simulink library "ddm"  (R2021b)
settings: Solver=VariableStepAuto  StartTime=0.0  StopTime=10.0  RelTol=1e-3
undefined symbols (not defined in the file or in its folder): ENUM_ADASACCSTA_ERROR, ENUM_ADASACCSTA_OFF, ENUM_ADASACCSTA_STANDBY, ENUM_ADASISASTA_OFF, ENUM_ALLOWMOV_ALLOWREADY, ENUM_APS, ENUM_BRKSTA_ERROR, ENUM_BRKSTA_OFF, ENUM_BRKSTA_ON, ENUM_BRKSW_INVALID, ENUM_BRKSW_OFF, ENUM_BRKSW_ON, ENUM_CHGPREACTERRSTA_OBCPRE, ENUM_DCDCFAULTSTA_ANYFAULTLV1, ENUM_DCDCFAULTSTA_ANYFAULTLV2, ENUM_DRIVETRAIN_AWD, ENUM_DRIVETRAIN_FWD, ENUM_DRIVETRAIN_RWD, ENUM_DRSEATSTA_INVALID, ENUM_EDUDRTSTA_NORMAL, ENUM_EPBSTA_APPLIED, ENUM_EPBSTA_RELEASED, ENUM_HVBATTREADYPRE_READY, ENUM_MCUWARN_LV0, ENUM_MCUWARN_LV1, ENUM_MCUWARN_LV2, ENUM_MCUWARN_LV3, ENUM_MCUWARN_NOERROR, ENUM_OBCFAULTSTA_ANYFAULT, ENUM_PAS_R2F2, ENUM_PDFAULT_BATTPDFAIL, ENUM_PDFAULT_DCDCDISABLE, ENUM_PDFAULT_MCUDISABLE, ENUM_PDFAULT_MCUDISCHRG, ENUM_POWERSTA_OFF, ENUM_POWERSTA_ON, ENUM_POWERSTA_READY, ENUM_POWERSTA_STANDBY, ENUM_PRESSINDI_LOW, ENUM_PUFAULT_BATTUPFAIL, ENUM_PUFAULT_DCDCENABLEFAIL, ENUM_PUFAULT_PRECHRGCHKFAIL, ENUM_PUFAULT_SAFETYCHKFAIL, ENUM_PUSTATE_COMPLETED, ENUM_PWRSTASW_OFF, ENUM_PWRSTASW_OFFA, ENUM_PWRSTASW_OFFCHVCHRG, ENUM_PWRSTASW_OFFCLVCHRG, ENUM_PWRSTASW_ON, ENUM_PWRSTASW_ONHVCHRG, ENUM_PWRSTASW_READY, ENUM_PWRSTASW_STANDBY, ENUM_RANGESTA_12IN, ENUM_SHIFTCOMMAND_D, ENUM_SHIFTCOMMAND_N, ENUM_SHIFTCOMMAND_P, ENUM_SHIFTCOMMAND_R, ENUM_VEHMALFUNLV_2ND, ENUM_VEHMALFUNLV_3RD, ENUM_VEHMALFUNLV_4TH ... (+835)
libraries: hcu_lib x750, $bdroot x12, simulink x5
(part 23 of 28)

== system ddm/DDM/DDM/VMC_DDM/ACC Acceleration Command Error/ACC Acceleration Command Error  ==
  note: Diagnostics and Fault Handling
  note: Fail Safe After Decision
  note: Release Condiction During Detection
  note: Release Condiction After Decision
  note: Test Pass Criteria
  note: Test Detection Criteria
  note: Fail Safe During Detection
  task_time_s : Inport
  VDDM_FCM2NoComCFS_flg : Inport  Port=2
  VDDM_FCM2RCErrCFS_flg : Inport  Port=3
  VDDM_FCM2CSErrCFS_flg : Inport  Port=4
  VVMC_ADASActive_flg : Inport  Port=5
  No_CAN_BUS_OFF : Inport  Port=6
  VPMM_PowerSta_enum : Inport  Port=7
  VINP_ACCRequireAccel_mps2 : Inport  Port=8
  VINP_ADASACCSta_enum : Inport  Port=9
  DTC_clear_request : Inport  Port=10
  Abs : Abs
  Abs1 : Abs
  Constant1 : Constant  Value=KDDM_ACCAccelCmdErrDet_mps2
  Constant10 : Constant  Value=ENUM_ADASACCSTA_OFF
  Constant11 : Constant  Value=KDDM_ACCAccelCmdErrPassSW_flg
  Constant12 : Constant  Value=ENUM_POWERSTA_OFF
  Constant13 : Constant  Value=ENUM_POWERSTA_STANDBY
  Constant{5,14,18,22} (4 alike) : Constant  Value=TRUE
  Constant{2,15..16,21,23} (5 alike) : Constant  Value=FALSE
  Constant3 : Constant  Value=KDDM_ACCAccelCmdErrDet_mps2
  Constant33 : Constant  Value=KDDM_ACCAccelCmdErrDetSW_flg
  Constant34 : Constant  Value=KDDM_ACCAccelCmdErrDTC_cnt
  Constant35 : Constant  Value=KDDM_ACCAccelCmdErrCFSSW_flg
  Constant36 : Constant  Value=KDDM_ACCAccelCmdErrDFSSW_flg
  Constant4 : Constant  Value=KDDM_ACCAccelCmdErrDetTO_ms
  Constant6 : Constant  Value=KDDM_ACCAccelCmdErrPassTO_ms
  Constant7 : Constant  Value=KDDM_ACCAccelCmdErrDTC_cnt
  Constant8 : Constant  Value=ENUM_ADASACCSTA_STANDBY
  Constant9 : Constant  Value=KDDM_ACCAccelCmdErrPassTO_ms
  DTC_Couter : hcu_lib/Basic_Blocks/DTC_Couter
  DTC_Info : hcu_lib/Basic_Blocks/DTC_Info
  Data Type Conversion1 : DataTypeConversion  OutDataTypeStr=uint8
  Equal1 : RelationalOperator  Operator=>  OutDataTypeStr=boolean  RndMeth=Simplest
  Equal2 : RelationalOperator  Operator=>  OutDataTypeStr=boolean  RndMeth=Simplest
  Equal3 : RelationalOperator  OutDataTypeStr=boolean  RndMeth=Simplest
  Equal{4..7} (4 alike) : RelationalOperator  Operator===  OutDataTypeStr=boolean  RndMeth=Simplest
  From1 : From  Commented=on  GotoTag=VDDM_ACCAccelCmdErrDFS_flg
  Gain : Gain  Gain=XX2KXX
  Gain1 : Gain  Gain=KXX2XX
  Goto7 : Goto  Commented=on  GotoTag=VDDM_EDriveSysErrVCUErr_flg
  Logical Operator{1,4,6,11,14,17..18,20} (8 alike) : Logic  Operator=NOT  AllPortsSameDT=off  OutDataTypeStr=boolean
  Logical Operator10 : Logic  Inputs=5  AllPortsSameDT=off  OutDataTypeStr=boolean
  Logical Operator12 : Logic  Operator=OR  Inputs=3  AllPortsSameDT=off  OutDataTypeStr=boolean
  Logical Operator{3,5,8,13,15} (5 alike) : Logic  AllPortsSameDT=off  OutDataTypeStr=boolean
  Logical Operator16 : Logic  Operator=OR  AllPortsSameDT=off  OutDataTypeStr=boolean
  Logical Operator19 : Logic  Inputs=3  AllPortsSameDT=off  OutDataTypeStr=boolean
  Logical Operator2 : Logic  Inputs=5  AllPortsSameDT=off  OutDataTypeStr=boolean
  Logical Operator25 : Logic  Operator=OR  Inputs=3  AllPortsSameDT=off  OutDataTypeStr=boolean
  Logical Operator7 : Logic  Operator=OR  Inputs=3  AllPortsSameDT=off  OutDataTypeStr=boolean
  Logical Operator9 : Logic  Operator=OR  AllPortsSameDT=off  OutDataTypeStr=boolean
  Relay : Relay  OnSwitchValue=ONE_INT  OffSwitchValue=ZERO_INT
  SR_Latch1 : hcu_lib/Basic_Blocks/SR_Latch
  SR_Latch4 : hcu_lib/Basic_Blocks/SR_Latch
  SR_Latch5 : hcu_lib/Basic_Blocks/SR_Latch
  Switch{,1..5} (6 alike) : Switch  Criteria=u2 ~= 0
  Terminator1 : Terminator
  Test Detection Criteria : hcu_lib/Basic_Blocks/Test Detection Criteria
  Timer1 : hcu_lib/Basic_Blocks/Timer
  Unit Delay2 : UnitDelay  SampleTime=-1  HasFrameUpgradeWarning=on
  VDDM_ACCAccelCmdErrCFS_flg : Outport
  VDDM_ACCAccelCmdErrDetDTC_raw32 : Outport  Port=2
  wires:
  Constant11/1 -> Logical Operator15/2
  DTC_Couter/1 -> SR_Latch5/1
  SR_Latch4/1 -> Logical Operator3/2
  Logical Operator25/1 -> Logical Operator15/1
  SR_Latch5/1 -> Logical Operator5/1
  Data Type Conversion1/1 -> [VDDM_ACCAccelCmdErrDTC_cnt]  "VDDM_ACCAccelCmdErrDTC_cnt"
  Constant36/1 -> Logical Operator3/1
  Relay/1 -> SR_Latch4/1
  [VDDM_ACCAccelCmdErrCFS_flg] -> Logical Operator7/2
  [VDDM_ACCAccelCmdErrDFSRls_flg] -> Logical Operator7/1
  [DTC_clear_request] -> Logical Operator25/1, Logical Operator14/1
  Constant33/1 -> Logical Operator19/2
  Logical Operator5/1 -> [VDDM_ACCAccelCmdErrCFS_flg]  "VDDM_ACCAccelCmdErrCFS_flg"
  Logical Operator3/1 -> [VDDM_ACCAccelCmdErrDFS_flg]
  [VDDM_ACCAccelCmdErrCFSRls_flg] -> Logical Operator25/3
  [VDDM_ACCAccelCmdErrPass_flg] -> Logical Operator25/2
  [VDDM_ACCAccelCmdErrDet_flg] -> Logical Operator19/1
  [DTC_clear_request] -> Logical Operator7/3
  Logical Operator16/1 -> SR_Latch5/2
  [DTC_clear_request] -> Logical Operator16/2
  Logical Operator14/1 -> Logical Operator19/3
  [VDDM_ACCAccelCmdErrCFSRls_flg] -> Logical Operator16/1
  [VDDM_ACCAccelCmdErrDTC_cnt] -> Relay/1
  Logical Operator15/1 -> DTC_Couter/2
  Logical Operator19/1 -> DTC_Couter/1
  Constant35/1 -> Logical Operator5/2
  Constant34/1 -> DTC_Couter/3
  DTC_Couter/2 -> Data Type Conversion1/1
  Logical Operator7/1 -> SR_Latch4/2
  DTC_Info/1 -> VDDM_ACCAccelCmdErrDetDTC_raw32/1  "VDDM_ACCAccelCmdErrDetDTC_raw32"
  [DTC_clear_request] -> DTC_Info/4
  [VDDM_ACCAccelCmdErrCFS_flg] -> DTC_Info/3
  [VDDM_ACCAccelCmdErrPass_flg] -> DTC_Info/2
  [VDDM_ACCAccelCmdErrDet_flg] -> DTC_Info/1
  [DTC_clear_request] -> Switch5/2
  Constant16/1 -> Switch5/1
  Switch5/1 -> Test Detection Criteria/1
  VINP_ADASACCSta_enum/1 -> [VINP_ADASACCSta_enum]
  [VDDM_ACCAccelCmdErrPass_flg] -> Logical Operator8/1
  Constant12/1 -> Equal6/2
  Equal5/1 -> Logical Operator9/2
  [VINP_ADASACCSta_enum] -> Equal4/1
  [VINP_ADASACCSta_enum] -> Equal5/1
  Constant13/1 -> Equal7/2
  Logical Operator8/1 -> Logical Operator12/1
  Equal4/1 -> Logical Operator9/1
  Equal6/1 -> Logical Operator13/1
  Logical Operator13/1 -> Logical Operator12/2
  Equal7/1 -> Logical Operator13/2
  Unit Delay2/1 -> Equal6/1
  Constant10/1 -> Equal4/2
  Logical Operator9/1 -> Logical Operator8/2
  Constant8/1 -> Equal5/2
  [VPMM_PowerSta_enum] -> Equal7/1
  [VPMM_PowerSta_enum] -> Unit Delay2/1
  [VDDM_FCM2NoComCFS_flg] -> Logical Operator1/1
  Abs1/1 -> Equal1/1
  [No_CAN_BUS_OFF] -> Logical Operator10/1
  [VDDM_FCM2CSErrCFS_flg] -> Logical Operator11/1
  Logical Operator10/1 -> Switch3/2
  Constant1/1 -> Equal1/2
  [VVMC_ADASActive_flg] -> Logical Operator10/5
  Equal1/1 -> Switch3/1
  Logical Operator4/1 -> Logical Operator10/3
  [VINP_ACCRequireAccel_mps2] -> Abs1/1
  Logical Operator11/1 -> Logical Operator10/4
  [VDDM_FCM2RCErrCFS_flg] -> Logical Operator4/1
  Logical Operator1/1 -> Logical Operator10/2
  Abs/1 -> Equal2/1
  VVMC_ADASActive_flg/1 -> [VVMC_ADASActive_flg]
  Equal2/1 -> Switch2/1
  Constant3/1 -> Equal2/2
  Constant9/1 -> Timer1/4
  Gain1/1 -> Timer1/3
  Test Detection Criteria/1 -> [VDDM_ACCAccelCmdErrDet_flg]  "VDDM_ACCAccelCmdErrDet_flg"
  Constant7/1 -> Test Detection Criteria/3
  Gain/1 -> Test Detection Criteria/4
  Constant4/1 -> Gain/1
  [task_time_s] -> Test Detection Criteria/2
  task_time_s/1 -> [task_time_s]  "task_time_s"
  Switch3/1 -> Logical Operator6/1, Timer1/2
  Constant5/1 -> Switch3/3
  Logical Operator20/1 -> Logical Operator2/4
  Logical Operator18/1 -> Logical Operator2/3
  Logical Operator17/1 -> Logical Operator2/2
  [VINP_ACCRequireAccel_mps2] -> Abs/1
  [VDDM_FCM2CSErrCFS_flg] -> Logical Operator20/1
  [VDDM_FCM2RCErrCFS_flg] -> Logical Operator18/1
  [VDDM_FCM2NoComCFS_flg] -> Logical Operator17/1
  [VVMC_ADASActive_flg] -> Logical Operator2/5
  VINP_ACCRequireAccel_mps2/1 -> [VINP_ACCRequireAccel_mps2]
  No_CAN_BUS_OFF/1 -> [No_CAN_BUS_OFF]
  VDDM_FCM2CSErrCFS_flg/1 -> [VDDM_FCM2CSErrCFS_flg]
  VPMM_PowerSta_enum/1 -> [VPMM_PowerSta_enum]
  VDDM_FCM2RCErrCFS_flg/1 -> [VDDM_FCM2RCErrCFS_flg]
  DTC_clear_request/1 -> [DTC_clear_request]
  VDDM_FCM2NoComCFS_flg/1 -> [VDDM_FCM2NoComCFS_flg]
  Timer1/1 -> Equal3/1
  Logical Operator12/1 -> Switch4/2
  Constant14/1 -> Switch4/1
  Constant2/1 -> Switch2/3
  Logical Operator6/1 -> Timer1/1
  Logical Operator2/1 -> Switch2/2
  [DTC_clear_request] -> Logical Operator12/3
  [VDDM_xxx_flg] -> SR_Latch1/2
  [No_CAN_BUS_OFF] -> Logical Operator2/1
  Switch4/1 -> [VDDM_ACCAccelCmdErrCFSRls_flg]  "VDDM_ACCAccelCmdErrCFSRls_flg"
  Constant6/1 -> Equal3/2
  [task_time_s] -> Gain1/1
  Equal3/1 -> SR_Latch1/1
  Constant15/1 -> Switch4/3
  [VDDM_ACCAccelCmdErrCFS_flg] -> VDDM_ACCAccelCmdErrCFS_flg/1
  From1/1 -> Terminator1/1
  SR_Latch1/1 -> [VDDM_ACCAccelCmdErrPass_flg]  "VDDM_ACCAccelCmdErrPass_flg"
  [VDDM_ACCAccelCmdErrPass_flg] -> Switch1/2
  [VDDM_ACCAccelCmdErrCFS_flg] -> Switch/2
  Constant18/1 -> Switch/1
  Switch/1 -> Goto7/1
  Constant21/1 -> Switch/3
  Switch1/1 -> [VDDM_ACCAccelCmdErrDFSRls_flg]
  Constant22/1 -> Switch1/1
  Constant23/1 -> Switch1/3
  Switch2/1 -> Switch5/3, [VDDM_xxx_flg]

== system ddm/DDM/DDM/VMC_DDM/ACC Malfunction /ACC Malfunction  ==
  note: Diagnostics and Fault Handling
  note: Fail Safe After Decision
  note: Release Condiction During Detection
  note: Release Condiction After Decision
  note: Test Pass Criteria
  note: Test Detection Criteria
  note: Fail Safe During Detection
  task_time_s : Inport
  VDDM_FCMACCSigErrCFS_flg : Inport  Port=2
  VDDM_ACCAccelCmdErrCFS_flg : Inport  Port=3
  VDDM_BMSSigErrCFS_flg : Inport  Port=4
  VDDM_FrMCUSigErrCFS_flg : Inport  Port=5
  VDDM_RrMCUSigErrCFS_flg : Inport  Port=6
  VDDM_CCUSigErrCFS_flg : Inport  Port=7
  VDDM_FCM2NoComCFS_flg : Inport  Port=8
  VDDM_FCM2RCErrCFS_flg : Inport  Port=9
  VDDM_FCM2CSErrCFS_flg : Inport  Port=10
  VDDM_FCM4NoComCFS_flg : Inport  Port=11
  VDDM_FCM4CSErrCFS_flg : Inport  Port=12
  VDDM_ZoneSCPNoComCFS_flg : Inport  Port=13
  VDDM_MCUR1NoComCFS_flg : Inport  Port=14
  VDDM_MCUR1RCErrCFS_flg : Inport  Port=15
  VDDM_MCUR1CSErrCFS_flg : Inport  Port=16
  VDDM_MCUF1NoComCFS_flg : Inport  Port=17
  VDDM_MCUF1RCErrCFS_flg : Inport  Port=18
  VDDM_MCUF1CSErrCFS_flg : Inport  Port=19
  VDDM_ESC7NoComCFS_flg : Inport  Port=20
  VDDM_ESC7RCErrCFS_flg : Inport  Port=21
  VDDM_ESC7CSErrCFS_flg : Inport  Port=22
  VDDM_ESC1NoComCFS_flg : Inport  Port=23
  VDDM_ESC1RCErrCFS_flg : Inport  Port=24
  VDDM_ESC1CSErrCFS_flg : Inport  Port=25
  VDDM_ESC5NoComCFS_flg : Inport  Port=26
  VDDM_ESC5RCErrCFS_flg : Inport  Port=27
  VDDM_ESC5CSErrCFS_flg : Inport  Port=28
  No_CAN1_BUS_OFF : Inport  Port=29
  No_CAN3_BUS_OFF : Inport  Port=30
  No_CAN4_BUS_OFF : Inport  Port=31
  VPMM_PowerSta_enum : Inport  Port=32
  VINP_ZoneSpdCtrlMode_enum : Inport  Port=33
  DTC_clear_request : Inport  Port=34
  Constant1 : Constant  Value=ENUM_POWERSTA_READY
  Constant10 : Constant  Value=ENUM_ZONESPDCTRLMODE_ACC
  Constant11 : Constant  Value=KDDM_ACCMalfuncPassSW_flg
  Constant12 : Constant  Value=ENUM_POWERSTA_OFF
  Constant13 : Constant  Value=ENUM_POWERSTA_STANDBY
  Constant{5,14,18,22} (4 alike) : Constant  Value=TRUE
  Constant{2,15..16,21,23} (5 alike) : Constant  Value=FALSE
  Constant3 : Constant  Value=ENUM_ZONESPDCTRLMODE_ACC
  Constant33 : Constant  Value=KDDM_ACCMalfuncDetSW_flg
  Constant34 : Constant  Value=KDDM_ACCMalfuncDTC_cnt
  Constant35 : Constant  Value=KDDM_ACCMalfuncCFSSW_flg
  Constant36 : Constant  Value=KDDM_ACCMalfuncDFSSW_flg
  Constant4 : Constant  Value=KDDM_ACCMalfuncDetTO_ms
  Constant6 : Constant  Value=KDDM_ACCMalfuncPassTO_ms
  Constant7 : Constant  Value=KDDM_ACCMalfuncDTC_cnt
  Constant8 : Constant  Value=ENUM_POWERSTA_READY
  Constant9 : Constant  Value=KDDM_ACCMalfuncPassTO_ms
  DTC_Couter : hcu_lib/Basic_Blocks/DTC_Couter
  DTC_Info : hcu_lib/Basic_Blocks/DTC_Info
  Data Type Conversion1 : DataTypeConversion  OutDataTypeStr=uint8
  Equal{1..2,4..7} (6 alike) : RelationalOperator  Operator===  OutDataTypeStr=boolean  RndMeth=Simplest
  Equal3 : RelationalOperator  OutDataTypeStr=boolean  RndMeth=Simplest
  From1 : From  Commented=on  GotoTag=VDDM_ACCMalfuncDFS_flg
  Gain : Gain  Gain=XX2KXX
  Gain1 : Gain  Gain=KXX2XX
  Goto7 : Goto  Commented=on  GotoTag=VDDM_EDriveSysErrVCUErr_flg
  Logical Operator1 : Logic  Inputs=5  AllPortsSameDT=off  OutDataTypeStr=boolean
  Logical Operator12 : Logic  Operator=OR  Inputs=3  AllPortsSameDT=off  OutDataTypeStr=boolean
  Logical Operator{3,5,13,15} (4 alike) : Logic  AllPortsSameDT=off  OutDataTypeStr=boolean
  Logical Operator14 : Logic  Operator=OR  Inputs=27  AllPortsSameDT=off  OutDataTypeStr=boolean
  Logical Operator19 : Logic  Inputs=3  AllPortsSameDT=off  OutDataTypeStr=boolean
  Logical Operator2 : Logic  Inputs=5  AllPortsSameDT=off  OutDataTypeStr=boolean
  Logical Operator25 : Logic  Operator=OR  Inputs=3  AllPortsSameDT=off  OutDataTypeStr=boolean
  Logical Operator4 : Logic  Operator=OR  Inputs=27  AllPortsSameDT=off  OutDataTypeStr=boolean
  Logical Operator6 : Logic  Operator=NOT  AllPortsSameDT=off  OutDataTypeStr=boolean
  Logical Operator7 : Logic  Operator=OR  Inputs=3  AllPortsSameDT=off  OutDataTypeStr=boolean
  Logical Operator8 : Logic  Operator=NOT  AllPortsSameDT=off  OutDataTypeStr=boolean
  Logical Operator9 : Logic  Operator=OR  AllPortsSameDT=off  OutDataTypeStr=boolean
  Relay : Relay  OnSwitchValue=ONE_INT  OffSwitchValue=ZERO_INT
  SR_Latch1 : hcu_lib/Basic_Blocks/SR_Latch
  SR_Latch4 : hcu_lib/Basic_Blocks/SR_Latch
  SR_Latch5 : hcu_lib/Basic_Blocks/SR_Latch
  Switch{,1..5} (6 alike) : Switch  Criteria=u2 ~= 0
  Terminator1 : Terminator
  Test Detection Criteria : hcu_lib/Basic_Blocks/Test Detection Criteria
  Timer1 : hcu_lib/Basic_Blocks/Timer
  Unit Delay2 : UnitDelay  SampleTime=-1  HasFrameUpgradeWarning=on
  VDDM_ACCMalfuncCFS_flg : Outport
  VDDM_ACCMalfuncDetDTC_raw32 : Outport  Port=2
  wires:
  [VDDM_ACCMalfuncDFSRls_flg] -> Logical Operator7/1
  Logical Operator8/1 -> Logical Operator19/3
  [DTC_clear_request] -> Logical Operator9/2
  Logical Operator5/1 -> [VDDM_ACCMalfuncCFS_flg]  "VDDM_ACCMalfuncCFS_flg"
  [DTC_clear_request] -> Logical Operator25/1, Logical Operator8/1
  [VDDM_ACCMalfuncCFSRls_flg] -> Logical Operator25/3
  Logical Operator9/1 -> SR_Latch5/2
  [VDDM_ACCMalfuncCFS_flg] -> Logical Operator7/2
  [VDDM_ACCMalfuncDTC_cnt] -> Relay/1
  [DTC_clear_request] -> Logical Operator7/3
  Constant35/1 -> Logical Operator5/2
  Constant33/1 -> Logical Operator19/2
  Logical Operator19/1 -> DTC_Couter/1
  SR_Latch5/1 -> Logical Operator5/1
  Relay/1 -> SR_Latch4/1
  Constant34/1 -> DTC_Couter/3
  Logical Operator25/1 -> Logical Operator15/1
  [VDDM_ACCMalfuncDet_flg] -> Logical Operator19/1
  Data Type Conversion1/1 -> [VDDM_ACCMalfuncDTC_cnt]  "VDDM_ACCMalfuncDTC_cnt"
  DTC_Couter/2 -> Data Type Conversion1/1
  Logical Operator7/1 -> SR_Latch4/2
  Constant36/1 -> Logical Operator3/1
  SR_Latch4/1 -> Logical Operator3/2
  [VDDM_ACCMalfuncCFSRls_flg] -> Logical Operator9/1
  Logical Operator15/1 -> DTC_Couter/2
  Logical Operator3/1 -> [VDDM_ACCMalfuncDFS_flg]
  [VDDM_ACCMalfuncPass_flg] -> Logical Operator25/2
  Constant11/1 -> Logical Operator15/2
  DTC_Couter/1 -> SR_Latch5/1
  DTC_Info/1 -> VDDM_ACCMalfuncDetDTC_raw32/1  "VDDM_ACCMalfuncDetDTC_raw32"
  [DTC_clear_request] -> DTC_Info/4
  [VDDM_ACCMalfuncCFS_flg] -> DTC_Info/3
  [VDDM_ACCMalfuncPass_flg] -> DTC_Info/2
  [VDDM_ACCMalfuncDet_flg] -> DTC_Info/1
  [DTC_clear_request] -> Switch5/2
  Constant16/1 -> Switch5/1
  Switch5/1 -> Test Detection Criteria/1
  [VDDM_ESC5NoComCFS_flg] -> Logical Operator4/25
  [VDDM_MCUF1RCErrCFS_flg] -> Logical Operator4/17
  [VDDM_ESC5RCErrCFS_flg] -> Logical Operator4/26
  [VDDM_MCUR1RCErrCFS_flg] -> Logical Operator4/14
  [VDDM_ESC5CSErrCFS_flg] -> Logical Operator4/27
  [VDDM_MCUF1NoComCFS_flg] -> Logical Operator4/16
  [VDDM_MCUR1CSErrCFS_flg] -> Logical Operator4/15
  [VDDM_ESC1RCErrCFS_flg] -> Logical Operator4/23
  [VDDM_ESC7NoComCFS_flg] -> Logical Operator4/19
  [VDDM_FrMCUSigErrCFS_flg] -> Logical Operator4/4
  [VDDM_MCUF1CSErrCFS_flg] -> Logical Operator4/18
  [VDDM_RrMCUSigErrCFS_flg] -> Logical Operator4/5
  [VDDM_ESC7RCErrCFS_flg] -> Logical Operator4/20
  [VDDM_FCM4CSErrCFS_flg] -> Logical Operator4/11
  [VDDM_ESC7CSErrCFS_flg] -> Logical Operator4/21
  [VDDM_MCUR1NoComCFS_flg] -> Logical Operator4/13
  [VDDM_ESC1NoComCFS_flg] -> Logical Operator4/22
  [VDDM_ESC1CSErrCFS_flg] -> Logical Operator4/24
  Logical Operator4/1 -> Switch3/1
  [VDDM_ACCAccelCmdErrCFS_flg] -> Logical Operator4/2
  [VDDM_BMSSigErrCFS_flg] -> Logical Operator4/3
  [VDDM_CCUSigErrCFS_flg] -> Logical Operator4/6
  [VDDM_FCM2NoComCFS_flg] -> Logical Operator4/7
  [VDDM_FCM2RCErrCFS_flg] -> Logical Operator4/8
  [VDDM_FCM4NoComCFS_flg] -> Logical Operator4/10
  [VDDM_FCM2CSErrCFS_flg] -> Logical Operator4/9
  [VDDM_ZoneSCPNoComCFS_flg] -> Logical Operator4/12
  [VDDM_FCMACCSigErrCFS_flg] -> Logical Operator4/1
  Logical Operator1/1 -> Switch3/2
  [No_CAN1_BUS_OFF] -> Logical Operator1/1
  [No_CAN3_BUS_OFF] -> Logical Operator1/2
  Equal4/1 -> Logical Operator1/5
  Equal5/1 -> Logical Operator1/4
  Constant8/1 -> Equal5/2
  Constant10/1 -> Equal4/2
  [VPMM_PowerSta_enum] -> Equal5/1
  [No_CAN4_BUS_OFF] -> Logical Operator1/3
  [VINP_ZoneSpdCtrlMode_enum] -> Equal4/1
  Equal1/1 -> Logical Operator2/5
  Constant3/1 -> Equal1/2
  [VINP_ZoneSpdCtrlMode_enum] -> Equal1/1
  [VPMM_PowerSta_enum] -> Equal2/1
  Constant1/1 -> Equal2/2
  Equal2/1 -> Logical Operator2/4
  [No_CAN4_BUS_OFF] -> Logical Operator2/3
  [No_CAN3_BUS_OFF] -> Logical Operator2/2
  Logical Operator14/1 -> Switch2/1
  [VDDM_ESC5CSErrCFS_flg] -> Logical Operator14/27
  [VDDM_ESC5RCErrCFS_flg] -> Logical Operator14/26
  [VDDM_ESC5NoComCFS_flg] -> Logical Operator14/25
  [VDDM_ESC1CSErrCFS_flg] -> Logical Operator14/24
  [VDDM_ESC1RCErrCFS_flg] -> Logical Operator14/23
  [VDDM_ESC1NoComCFS_flg] -> Logical Operator14/22
  [VDDM_ESC7CSErrCFS_flg] -> Logical Operator14/21
  [VDDM_ESC7RCErrCFS_flg] -> Logical Operator14/20
  [VDDM_ESC7NoComCFS_flg] -> Logical Operator14/19
  [VDDM_MCUF1CSErrCFS_flg] -> Logical Operator14/18
  [VDDM_MCUF1RCErrCFS_flg] -> Logical Operator14/17
  [VDDM_MCUF1NoComCFS_flg] -> Logical Operator14/16
  [VDDM_MCUR1CSErrCFS_flg] -> Logical Operator14/15
  [VDDM_MCUR1RCErrCFS_flg] -> Logical Operator14/14
  [VDDM_MCUR1NoComCFS_flg] -> Logical Operator14/13
  [VDDM_ZoneSCPNoComCFS_flg] -> Logical Operator14/12
  [VDDM_FCM4CSErrCFS_flg] -> Logical Operator14/11
  [VDDM_FCM4NoComCFS_flg] -> Logical Operator14/10
  [VDDM_FCM2CSErrCFS_flg] -> Logical Operator14/9
  [VDDM_FCM2RCErrCFS_flg] -> Logical Operator14/8
  [VDDM_FCM2NoComCFS_flg] -> Logical Operator14/7
  [VDDM_CCUSigErrCFS_flg] -> Logical Operator14/6
  [VDDM_RrMCUSigErrCFS_flg] -> Logical Operator14/5
  [VDDM_FrMCUSigErrCFS_flg] -> Logical Operator14/4
  [VDDM_BMSSigErrCFS_flg] -> Logical Operator14/3
  [VDDM_ACCAccelCmdErrCFS_flg] -> Logical Operator14/2
  [VDDM_FCMACCSigErrCFS_flg] -> Logical Operator14/1
  VDDM_ESC5RCErrCFS_flg/1 -> [VDDM_ESC5RCErrCFS_flg]
  VDDM_ACCAccelCmdErrCFS_flg/1 -> [VDDM_ACCAccelCmdErrCFS_flg]
  VDDM_ESC5CSErrCFS_flg/1 -> [VDDM_ESC5CSErrCFS_flg]
  VDDM_ESC5NoComCFS_flg/1 -> [VDDM_ESC5NoComCFS_flg]
  VDDM_ZoneSCPNoComCFS_flg/1 -> [VDDM_ZoneSCPNoComCFS_flg]
  task_time_s/1 -> [task_time_s]  "task_time_s"
  VINP_ZoneSpdCtrlMode_enum/1 -> [VINP_ZoneSpdCtrlMode_enum]
  No_CAN3_BUS_OFF/1 -> [No_CAN3_BUS_OFF]
  No_CAN1_BUS_OFF/1 -> [No_CAN1_BUS_OFF]
  VDDM_BMSSigErrCFS_flg/1 -> [VDDM_BMSSigErrCFS_flg]
  VDDM_ESC7NoComCFS_flg/1 -> [VDDM_ESC7NoComCFS_flg]
  VDDM_FCMACCSigErrCFS_flg/1 -> [VDDM_FCMACCSigErrCFS_flg]
  VDDM_ESC7CSErrCFS_flg/1 -> [VDDM_ESC7CSErrCFS_flg]
  VPMM_PowerSta_enum/1 -> [VPMM_PowerSta_enum]
  No_CAN4_BUS_OFF/1 -> [No_CAN4_BUS_OFF]
  VDDM_ESC7RCErrCFS_flg/1 -> [VDDM_ESC7RCErrCFS_flg]
  VDDM_RrMCUSigErrCFS_flg/1 -> [VDDM_RrMCUSigErrCFS_flg]
  VDDM_CCUSigErrCFS_flg/1 -> [VDDM_CCUSigErrCFS_flg]
  VDDM_FrMCUSigErrCFS_flg/1 -> [VDDM_FrMCUSigErrCFS_flg]
  VDDM_MCUF1RCErrCFS_flg/1 -> [VDDM_MCUF1RCErrCFS_flg]
  VDDM_ESC1NoComCFS_flg/1 -> [VDDM_ESC1NoComCFS_flg]
  DTC_clear_request/1 -> [DTC_clear_request]
  VDDM_FCM4CSErrCFS_flg/1 -> [VDDM_FCM4CSErrCFS_flg]
  VDDM_FCM4NoComCFS_flg/1 -> [VDDM_FCM4NoComCFS_flg]
  VDDM_FCM2CSErrCFS_flg/1 -> [VDDM_FCM2CSErrCFS_flg]
  VDDM_FCM2NoComCFS_flg/1 -> [VDDM_FCM2NoComCFS_flg]
  VDDM_FCM2RCErrCFS_flg/1 -> [VDDM_FCM2RCErrCFS_flg]
  VDDM_MCUR1RCErrCFS_flg/1 -> [VDDM_MCUR1RCErrCFS_flg]
  VDDM_MCUR1CSErrCFS_flg/1 -> [VDDM_MCUR1CSErrCFS_flg]
  VDDM_ESC1RCErrCFS_flg/1 -> [VDDM_ESC1RCErrCFS_flg]
  VDDM_ESC1CSErrCFS_flg/1 -> [VDDM_ESC1CSErrCFS_flg]
  VDDM_MCUF1CSErrCFS_flg/1 -> [VDDM_MCUF1CSErrCFS_flg]
  VDDM_MCUF1NoComCFS_flg/1 -> [VDDM_MCUF1NoComCFS_flg]
  VDDM_MCUR1NoComCFS_flg/1 -> [VDDM_MCUR1NoComCFS_flg]
  [VDDM_ACCMalfuncPass_flg] -> Logical Operator12/1
  Constant12/1 -> Equal6/2
  Constant13/1 -> Equal7/2
  Equal6/1 -> Logical Operator13/1
  Logical Operator13/1 -> Logical Operator12/2
  Equal7/1 -> Logical Operator13/2
  Unit Delay2/1 -> Equal6/1
  [VPMM_PowerSta_enum] -> Equal7/1
  [VPMM_PowerSta_enum] -> Unit Delay2/1
  Constant9/1 -> Timer1/4
  Gain1/1 -> Timer1/3
  Test Detection Criteria/1 -> [VDDM_ACCMalfuncDet_flg]  "VDDM_ACCMalfuncDet_flg"
  Constant7/1 -> Test Detection Criteria/3
  Gain/1 -> Test Detection Criteria/4
  Constant4/1 -> Gain/1
  [task_time_s] -> Test Detection Criteria/2
  Switch3/1 -> Logical Operator6/1, Timer1/2
  Constant5/1 -> Switch3/3
  Timer1/1 -> Equal3/1
  Logical Operator12/1 -> Switch4/2
  Constant14/1 -> Switch4/1
  Constant2/1 -> Switch2/3
  Logical Operator6/1 -> Timer1/1
  Logical Operator2/1 -> Switch2/2
  [DTC_clear_request] -> Logical Operator12/3
  [VDDM_xxx_flg] -> SR_Latch1/2
  [No_CAN1_BUS_OFF] -> Logical Operator2/1
  Switch4/1 -> [VDDM_ACCMalfuncCFSRls_flg]  "VDDM_ACCMalfuncCFSRls_flg"
  Constant6/1 -> Equal3/2
  [task_time_s] -> Gain1/1
  Equal3/1 -> SR_Latch1/1
  Constant15/1 -> Switch4/3
  [VDDM_ACCMalfuncCFS_flg] -> VDDM_ACCMalfuncCFS_flg/1
  From1/1 -> Terminator1/1
  SR_Latch1/1 -> [VDDM_ACCMalfuncPass_flg]  "VDDM_ACCMalfuncPass_flg"
  [VDDM_ACCMalfuncPass_flg] -> Switch1/2
  [VDDM_ACCMalfuncCFS_flg] -> Switch/2
  Constant18/1 -> Switch/1
  Switch/1 -> Goto7/1
  Constant21/1 -> Switch/3
  Switch1/1 -> [VDDM_ACCMalfuncDFSRls_flg]
  Constant22/1 -> Switch1/1
  Constant23/1 -> Switch1/3
  Switch2/1 -> Switch5/3, [VDDM_xxx_flg]

== system ddm/DDM/DDM/VMC_DDM/BMS Signal Error /BMS Signal Error  ==
  note: Diagnostics and Fault Handling
  note: Fail Safe After Decision
  note: Release Condiction During Detection
  note: Release Condiction After Decision
  note: Test Pass Criteria
  note: Test Detection Criteria
  note: Fail Safe During Detection
  task_time_s : Inport
  VDDM_C3BMS6LCCFS_flg : Inport  Port=2
  VDDM_C3BMS6RCCFS_flg : Inport  Port=3
  VDDM_C3BMS6CSCFS_flg : Inport  Port=4
  No_CAN_BUS_OFF : Inport  Port=5
  VPMM_PowerSta_enum : Inport  Port=6
  VINP_BMSWarn8_flg : Inport  Port=7
  VINP_BMSWarn7_flg : Inport  Port=8
  VINP_BMSWarn6_flg : Inport  Port=9
  VINP_BMSWarn5_flg : Inport  Port=10
  VINP_BMSWarn4_flg : Inport  Port=11
  DTC_clear_request : Inport  Port=12
  Constant : Constant  Value=ENUM_POWERSTA_OFF
  Constant1 : Constant  Value=ENUM_POWERSTA_OFF
  Constant11 : Constant  Value=KDDM_BMSSigErrPassSW_flg
  Constant12 : Constant  Value=ENUM_POWERSTA_OFF
  Constant13 : Constant  Value=ENUM_POWERSTA_STANDBY
  Constant{5,14,18,22} (4 alike) : Constant  Value=TRUE
  Constant{2..3,15,21,23} (5 alike) : Constant  Value=FALSE
  Constant33 : Constant  Value=KDDM_BMSSigErrDetSW_flg
  Constant34 : Constant  Value=KDDM_BMSSigErrDTC_cnt
  Constant35 : Constant  Value=KDDM_BMSSigErrCFSSW_flg
  Constant36 : Constant  Value=KDDM_BMSSigErrDFSSW_flg
  Constant4 : Constant  Value=KDDM_BMSSigErrDetTO_ms
  Constant6 : Constant  Value=KDDM_BMSSigErrPassTO_ms
  Constant7 : Constant  Value=KDDM_BMSSigErrDTC_cnt
  Constant9 : Constant  Value=KDDM_BMSSigErrPassTO_ms
  DTC_Couter : hcu_lib/Basic_Blocks/DTC_Couter
  DTC_Info : hcu_lib/Basic_Blocks/DTC_Info
  Data Type Conversion1 : DataTypeConversion  OutDataTypeStr=uint8
  Equal : RelationalOperator  Operator=~=  OutDataTypeStr=boolean  RndMeth=Simplest
  Equal1 : RelationalOperator  Operator=~=  OutDataTypeStr=boolean  RndMeth=Simplest
  Equal3 : RelationalOperator  OutDataTypeStr=boolean  RndMeth=Simplest
  Equal6 : RelationalOperator  Operator===  OutDataTypeStr=boolean  RndMeth=Simplest
  Equal7 : RelationalOperator  Operator===  OutDataTypeStr=boolean  RndMeth=Simplest
  From1 : From  Commented=on  GotoTag=VDDM_BMSSigErrDFS_flg
  Gain : Gain  Gain=XX2KXX
  Gain1 : Gain  Gain=KXX2XX
  Goto7 : Goto  Commented=on  GotoTag=VDDM_EDriveSysErrVCUErr_flg
  Logical Operator{1,6,17..18,20..22,24} (8 alike) : Logic  Operator=NOT  AllPortsSameDT=off  OutDataTypeStr=boolean
  Logical Operator10 : Logic  Operator=OR  AllPortsSameDT=off  OutDataTypeStr=boolean
  Logical Operator{3,5,9,15} (4 alike) : Logic  AllPortsSameDT=off  OutDataTypeStr=boolean
  Logical Operator16 : Logic  Operator=OR  Inputs=5  AllPortsSameDT=off  OutDataTypeStr=boolean
  Logical Operator19 : Logic  Inputs=3  AllPortsSameDT=off  OutDataTypeStr=boolean
  Logical Operator2 : Logic  Inputs=5  AllPortsSameDT=off  OutDataTypeStr=boolean
  Logical Operator23 : Logic  Inputs=5  AllPortsSameDT=off  OutDataTypeStr=boolean
  Logical Operator25 : Logic  Operator=OR  Inputs=3  AllPortsSameDT=off  OutDataTypeStr=boolean
  Logical Operator4 : Logic  Operator=OR  Inputs=5  AllPortsSameDT=off  OutDataTypeStr=boolean
  Logical Operator7 : Logic  Operator=OR  Inputs=3  AllPortsSameDT=off  OutDataTypeStr=boolean
  Logical Operator8 : Logic  Operator=OR  Inputs=3  AllPortsSameDT=off  OutDataTypeStr=boolean
  Relay : Relay  OnSwitchValue=ONE_INT  OffSwitchValue=ZERO_INT
  SR_Latch1 : hcu_lib/Basic_Blocks/SR_Latch
  SR_Latch4 : hcu_lib/Basic_Blocks/SR_Latch
  SR_Latch5 : hcu_lib/Basic_Blocks/SR_Latch
  Switch{,1..5} (6 alike) : Switch  Criteria=u2 ~= 0
  Terminator1 : Terminator
  Test Detection Criteria : hcu_lib/Basic_Blocks/Test Detection Criteria
  Timer1 : hcu_lib/Basic_Blocks/Timer
  Unit Delay2 : UnitDelay  SampleTime=-1  HasFrameUpgradeWarning=on
  VDDM_BMSSigErrCFS_flg : Outport
  VDDM_BMSSigErrDetDTC_raw32 : Outport  Port=2
  wires:
  Logical Operator25/1 -> Logical Operator15/1
  SR_Latch4/1 -> Logical Operator3/2
  [VDDM_BMSSigErrPass_flg] -> Logical Operator25/2
  Logical Operator1/1 -> Logical Operator19/3
  Logical Operator7/1 -> SR_Latch4/2
  [VDDM_BMSSigErrCFSRls_flg] -> Logical Operator25/3
  [DTC_clear_request] -> Logical Operator7/3
  [VDDM_BMSSigErrDTC_cnt] -> Relay/1
  Relay/1 -> SR_Latch4/1
  Constant34/1 -> DTC_Couter/3
  Constant33/1 -> Logical Operator19/2
  [VDDM_BMSSigErrDFSRls_flg] -> Logical Operator7/1
  Data Type Conversion1/1 -> [VDDM_BMSSigErrDTC_cnt]
  Logical Operator19/1 -> DTC_Couter/1
  [VDDM_BMSSigErrCFSRls_flg] -> Logical Operator10/1
  DTC_Couter/2 -> Data Type Conversion1/1
  DTC_Couter/1 -> SR_Latch5/1
  Logical Operator5/1 -> [VDDM_BMSSigErrCFS_flg]  "VDDM_BMSSigErrCFS_flg"
  Constant36/1 -> Logical Operator3/1
  Logical Operator10/1 -> SR_Latch5/2
  [DTC_clear_request] -> Logical Operator10/2
  [DTC_clear_request] -> Logical Operator25/1, Logical Operator1/1
  [VDDM_BMSSigErrCFS_flg] -> Logical Operator7/2
  Constant35/1 -> Logical Operator5/2
  SR_Latch5/1 -> Logical Operator5/1
  Logical Operator15/1 -> DTC_Couter/2
  [VDDM_BMSSigErrDet_flg] -> Logical Operator19/1
  Constant11/1 -> Logical Operator15/2
  Logical Operator3/1 -> [VDDM_BMSSigErrDFS_flg]
  DTC_Info/1 -> VDDM_BMSSigErrDetDTC_raw32/1  "VDDM_BMSSigErrDetDTC_raw32"
  [DTC_clear_request] -> DTC_Info/4
  [VDDM_BMSSigErrCFS_flg] -> DTC_Info/3
  [VDDM_BMSSigErrPass_flg] -> DTC_Info/2
  [VDDM_BMSSigErrDet_flg] -> DTC_Info/1
  Switch5/1 -> Test Detection Criteria/1
  [DTC_clear_request] -> Switch5/2
  Constant3/1 -> Switch5/1
  Constant9/1 -> Timer1/4
  Gain1/1 -> Timer1/3
  Test Detection Criteria/1 -> [VDDM_BMSSigErrDet_flg]  "VDDM_BMSSigErrDet_flg"
  Constant7/1 -> Test Detection Criteria/3
  Gain/1 -> Test Detection Criteria/4
  Constant4/1 -> Gain/1
  [task_time_s] -> Test Detection Criteria/2
  task_time_s/1 -> [task_time_s]  "task_time_s"
  [VINP_BMSWarn8_flg] -> Logical Operator4/1
  [VINP_BMSWarn6_flg] -> Logical Operator4/3
  [VINP_BMSWarn4_flg] -> Logical Operator4/5
  Switch3/1 -> Logical Operator6/1, Timer1/2
  Constant1/1 -> Equal1/2
  [No_CAN_BUS_OFF] -> Logical Operator23/1
  [VINP_BMSWarn5_flg] -> Logical Operator4/4
  [VDDM_C3BMS6CSCFS_flg] -> Logical Operator24/1
  Logical Operator21/1 -> Logical Operator23/2
  Logical Operator24/1 -> Logical Operator23/4
  [VINP_BMSWarn7_flg] -> Logical Operator4/2
  [VDDM_C3BMS6RCCFS_flg] -> Logical Operator22/1
  Equal1/1 -> Logical Operator23/5
  Constant5/1 -> Switch3/3
  Logical Operator23/1 -> Switch3/2
  [VPMM_PowerSta_enum] -> Equal1/1
  Logical Operator4/1 -> Switch3/1
  [VDDM_C3BMS6LCCFS_flg] -> Logical Operator21/1
  Logical Operator22/1 -> Logical Operator23/3
  Logical Operator20/1 -> Logical Operator2/4
  Logical Operator18/1 -> Logical Operator2/3
  Logical Operator17/1 -> Logical Operator2/2
  [VINP_BMSWarn4_flg] -> Logical Operator16/5
  [VINP_BMSWarn5_flg] -> Logical Operator16/4
  [VINP_BMSWarn6_flg] -> Logical Operator16/3
  [VINP_BMSWarn7_flg] -> Logical Operator16/2
  [VINP_BMSWarn8_flg] -> Logical Operator16/1
  Logical Operator16/1 -> Switch2/1
  [VDDM_C3BMS6CSCFS_flg] -> Logical Operator20/1
  [VDDM_C3BMS6RCCFS_flg] -> Logical Operator18/1
  [VDDM_C3BMS6LCCFS_flg] -> Logical Operator17/1
  Equal/1 -> Logical Operator2/5
  VINP_BMSWarn8_flg/1 -> [VINP_BMSWarn8_flg]
  No_CAN_BUS_OFF/1 -> [No_CAN_BUS_OFF]
  VDDM_C3BMS6CSCFS_flg/1 -> [VDDM_C3BMS6CSCFS_flg]
  VINP_BMSWarn7_flg/1 -> [VINP_BMSWarn7_flg]
  VPMM_PowerSta_enum/1 -> [VPMM_PowerSta_enum]
  VDDM_C3BMS6RCCFS_flg/1 -> [VDDM_C3BMS6RCCFS_flg]
  DTC_clear_request/1 -> [DTC_clear_request]
  VDDM_C3BMS6LCCFS_flg/1 -> [VDDM_C3BMS6LCCFS_flg]
  VINP_BMSWarn4_flg/1 -> [VINP_BMSWarn4_flg]
  VINP_BMSWarn5_flg/1 -> [VINP_BMSWarn5_flg]
  VINP_BMSWarn6_flg/1 -> [VINP_BMSWarn6_flg]
  Timer1/1 -> Equal3/1
  [VPMM_PowerSta_enum] -> Equal/1
  Logical Operator8/1 -> Switch4/2
  [VPMM_PowerSta_enum] -> Equal7/1
  Constant14/1 -> Switch4/1
  Constant2/1 -> Switch2/3
  Constant12/1 -> Equal6/2
  Unit Delay2/1 -> Equal6/1
  Constant/1 -> Equal/2
  Constant13/1 -> Equal7/2
  Logical Operator6/1 -> Timer1/1
  Logical Operator2/1 -> Switch2/2
  [DTC_clear_request] -> Logical Operator8/3
  [VDDM_xxx_flg] -> SR_Latch1/2
  [VDDM_BMSSigErrPass_flg] -> Logical Operator8/1
  [No_CAN_BUS_OFF] -> Logical Operator2/1
  Switch4/1 -> [VDDM_BMSSigErrCFSRls_flg]  "VDDM_BMSSigErrCFSRls_flg"
  Logical Operator9/1 -> Logical Operator8/2
  [VPMM_PowerSta_enum] -> Unit Delay2/1
  Constant6/1 -> Equal3/2
  Equal7/1 -> Logical Operator9/2
  Equal6/1 -> Logical Operator9/1
  [task_time_s] -> Gain1/1
  Equal3/1 -> SR_Latch1/1
  Constant15/1 -> Switch4/3
  [VDDM_BMSSigErrCFS_flg] -> VDDM_BMSSigErrCFS_flg/1
  From1/1 -> Terminator1/1
  SR_Latch1/1 -> [VDDM_BMSSigErrPass_flg]  "VDDM_BMSSigErrPass_flg"
  [VDDM_BMSSigErrPass_flg] -> Switch1/2
  [VDDM_BMSSigErrCFS_flg] -> Switch/2
  Constant18/1 -> Switch/1
  Switch/1 -> Goto7/1
  Constant21/1 -> Switch/3
  Switch1/1 -> [VDDM_BMSSigErrDFSRls_flg]
  Constant22/1 -> Switch1/1
  Constant23/1 -> Switch1/3
  Switch2/1 -> Switch5/3, [VDDM_xxx_flg]

== system ddm/DDM/DDM/VMC_DDM/CC Malfunction /CC Malfunction  ==
  note: Diagnostics and Fault Handling
  note: Fail Safe After Decision
  note: Release Condiction During Detection
  note: Release Condiction After Decision
  note: Test Pass Criteria
  note: Test Detection Criteria
  note: Fail Safe During Detection
  task_time_s : Inport
  VDDM_BMSSigErrCFS_flg : Inport  Port=2
  VDDM_FrMCUSigErrCFS_flg : Inport  Port=3
  VDDM_RrMCUSigErrCFS_flg : Inport  Port=4
  VDDM_CCUSigErrCFS_flg : Inport  Port=5
  VDDM_ZoneSCPNoComCFS_flg : Inport  Port=6
  VDDM_MCUR1NoComCFS_flg : Inport  Port=7
  VDDM_MCUR1RCErrCFS_flg : Inport  Port=8
  VDDM_MCUR1CSErrCFS_flg : Inport  Port=9
  VDDM_MCUF1NoComCFS_flg : Inport  Port=10
  VDDM_MCUF1RCErrCFS_flg : Inport  Port=11
  VDDM_MCUF1CSErrCFS_flg : Inport  Port=12
  VDDM_ESC7NoComCFS_flg : Inport  Port=13
  VDDM_ESC7RCErrCFS_flg : Inport  Port=14
  VDDM_ESC7CSErrCFS_flg : Inport  Port=15
  VDDM_ESC1NoComCFS_flg : Inport  Port=16
  VDDM_ESC1RCErrCFS_flg : Inport  Port=17
  VDDM_ESC1CSErrCFS_flg : Inport  Port=18
  VDDM_ESC5NoComCFS_flg : Inport  Port=19
  VDDM_ESC5RCErrCFS_flg : Inport  Port=20
  VDDM_ESC5CSErrCFS_flg : Inport  Port=21
  No_CAN1_BUS_OFF : Inport  Port=22
  No_CAN3_BUS_OFF : Inport  Port=23
  No_CAN4_BUS_OFF : Inport  Port=24
  VPMM_PowerSta_enum : Inport  Port=25
  VINP_ZoneSpdCtrlMode_enum : Inport  Port=26
  DTC_clear_request : Inport  Port=27
  Constant1 : Constant  Value=ENUM_POWERSTA_READY
  Constant10 : Constant  Value=ENUM_ZONESPDCTRLMODE_CC
  Constant11 : Constant  Value=KDDM_CCMalfuncPassSW_flg
  Constant12 : Constant  Value=ENUM_POWERSTA_OFF
  Constant13 : Constant  Value=ENUM_POWERSTA_STANDBY
  Constant{5,14,18,22} (4 alike) : Constant  Value=TRUE
  Constant{2,15..16,21,23} (5 alike) : Constant  Value=FALSE
  Constant3 : Constant  Value=ENUM_ZONESPDCTRLMODE_CC
  Constant33 : Constant  Value=KDDM_CCMalfuncDetSW_flg
  Constant34 : Constant  Value=KDDM_CCMalfuncDTC_cnt
  Constant35 : Constant  Value=KDDM_CCMalfuncCFSSW_flg
  Constant36 : Constant  Value=KDDM_CCMalfuncDFSSW_flg
  Constant4 : Constant  Value=KDDM_CCMalfuncDetTO_ms
  Constant6 : Constant  Value=KDDM_CCMalfuncPassTO_ms
  Constant7 : Constant  Value=KDDM_CCMalfuncDTC_cnt
  Constant8 : Constant  Value=ENUM_POWERSTA_READY
  Constant9 : Constant  Value=KDDM_CCMalfuncPassTO_ms
  DTC_Couter : hcu_lib/Basic_Blocks/DTC_Couter
  DTC_Info : hcu_lib/Basic_Blocks/DTC_Info
  Data Type Conversion1 : DataTypeConversion  OutDataTypeStr=uint8
  Equal{1..2,4..7} (6 alike) : RelationalOperator  Operator===  OutDataTypeStr=boolean  RndMeth=Simplest
  Equal3 : RelationalOperator  OutDataTypeStr=boolean  RndMeth=Simplest
  From1 : From  Commented=on  GotoTag=VDDM_CCMalfuncDFS_flg
  Gain : Gain  Gain=XX2KXX
  Gain1 : Gain  Gain=KXX2XX
  Goto7 : Goto  Commented=on  GotoTag=VDDM_EDriveSysErrVCUErr_flg
  Logical Operator1 : Logic  Inputs=5  AllPortsSameDT=off  OutDataTypeStr=boolean
  Logical Operator12 : Logic  Operator=OR  Inputs=3  AllPortsSameDT=off  OutDataTypeStr=boolean
  Logical Operator{3,5,13,15} (4 alike) : Logic  AllPortsSameDT=off  OutDataTypeStr=boolean
  Logical Operator14 : Logic  Operator=OR  Inputs=20  AllPortsSameDT=off  OutDataTypeStr=boolean
  Logical Operator19 : Logic  Inputs=3  AllPortsSameDT=off  OutDataTypeStr=boolean
  Logical Operator2 : Logic  Inputs=5  AllPortsSameDT=off  OutDataTypeStr=boolean
  Logical Operator25 : Logic  Operator=OR  Inputs=3  AllPortsSameDT=off  OutDataTypeStr=boolean
  Logical Operator4 : Logic  Operator=OR  Inputs=20  AllPortsSameDT=off  OutDataTypeStr=boolean
  Logical Operator6 : Logic  Operator=NOT  AllPortsSameDT=off  OutDataTypeStr=boolean
  Logical Operator7 : Logic  Operator=OR  Inputs=3  AllPortsSameDT=off  OutDataTypeStr=boolean
  Logical Operator8 : Logic  Operator=NOT  AllPortsSameDT=off  OutDataTypeStr=boolean
  Logical Operator9 : Logic  Operator=OR  AllPortsSameDT=off  OutDataTypeStr=boolean
  Relay : Relay  OnSwitchValue=ONE_INT  OffSwitchValue=ZERO_INT
  SR_Latch1 : hcu_lib/Basic_Blocks/SR_Latch
  SR_Latch4 : hcu_lib/Basic_Blocks/SR_Latch
  SR_Latch5 : hcu_lib/Basic_Blocks/SR_Latch
  Switch{,1..5} (6 alike) : Switch  Criteria=u2 ~= 0
  Terminator1 : Terminator
  Test Detection Criteria : hcu_lib/Basic_Blocks/Test Detection Criteria
  Timer1 : hcu_lib/Basic_Blocks/Timer
  Unit Delay2 : UnitDelay  SampleTime=-1  HasFrameUpgradeWarning=on
  VDDM_CCMalfuncCFS_flg : Outport
  VDDM_CCMalfuncDetDTC_raw32 : Outport  Port=2
  wires:
  Logical Operator9/1 -> SR_Latch5/2
  Logical Operator3/1 -> [VDDM_CCMalfuncDFS_flg]
  Constant33/1 -> Logical Operator19/2
  [VDDM_CCMalfuncCFS_flg] -> Logical Operator7/2
  [VDDM_CCMalfuncDet_flg] -> Logical Operator19/1
  DTC_Couter/1 -> SR_Latch5/1
  [VDDM_CCMalfuncPass_flg] -> Logical Operator25/2
  [VDDM_CCMalfuncCFSRls_flg] -> Logical Operator25/3
  [VDDM_CCMalfuncCFSRls_flg] -> Logical Operator9/1
  Constant11/1 -> Logical Operator15/2
  DTC_Couter/2 -> Data Type Conversion1/1
  [VDDM_CCMalfuncDTC_cnt] -> Relay/1
  Constant34/1 -> DTC_Couter/3
  Logical Operator25/1 -> Logical Operator15/1
  Logical Operator8/1 -> Logical Operator19/3
  Constant35/1 -> Logical Operator5/2
  [DTC_clear_request] -> Logical Operator25/1, Logical Operator8/1
  SR_Latch5/1 -> Logical Operator5/1
  [DTC_clear_request] -> Logical Operator7/3
  [VDDM_CCMalfuncDFSRls_flg] -> Logical Operator7/1
  SR_Latch4/1 -> Logical Operator3/2
  Constant36/1 -> Logical Operator3/1
  Logical Operator15/1 -> DTC_Couter/2
  Logical Operator5/1 -> [VDDM_CCMalfuncCFS_flg]  "VDDM_CCMalfuncCFS_flg"
  Logical Operator19/1 -> DTC_Couter/1
  Data Type Conversion1/1 -> [VDDM_CCMalfuncDTC_cnt]  "VDDM_CCMalfuncDTC_cnt"
  Relay/1 -> SR_Latch4/1
  Logical Operator7/1 -> SR_Latch4/2
  [DTC_clear_request] -> Logical Operator9/2
  DTC_Info/1 -> VDDM_CCMalfuncDetDTC_raw32/1  "VDDM_CCMalfuncDetDTC_raw32"
  [DTC_clear_request] -> DTC_Info/4
  [VDDM_CCMalfuncCFS_flg] -> DTC_Info/3
  [VDDM_CCMalfuncPass_flg] -> DTC_Info/2
  [VDDM_CCMalfuncDet_flg] -> DTC_Info/1
  Switch2/1 -> Switch5/3, [VDDM_xxx_flg]
  Switch5/1 -> Test Detection Criteria/1
  Constant16/1 -> Switch5/1
  [DTC_clear_request] -> Switch5/2
  [VDDM_ESC5CSErrCFS_flg] -> Logical Operator4/20
  [VDDM_MCUR1CSErrCFS_flg] -> Logical Operator4/8
  [VDDM_ESC5NoComCFS_flg] -> Logical Operator4/18
  Logical Operator4/1 -> Switch3/1
  [VDDM_CCUSigErrCFS_flg] -> Logical Operator4/4
  [VDDM_MCUR1RCErrCFS_flg] -> Logical Operator4/7
  [VDDM_ESC1CSErrCFS_flg] -> Logical Operator4/17
  [VDDM_MCUF1NoComCFS_flg] -> Logical Operator4/9
  [VDDM_MCUR1NoComCFS_flg] -> Logical Operator4/6
  [VDDM_MCUF1CSErrCFS_flg] -> Logical Operator4/11
  [VDDM_MCUF1RCErrCFS_flg] -> Logical Operator4/10
  [VDDM_ESC7NoComCFS_flg] -> Logical Operator4/12
  [VDDM_ESC1NoComCFS_flg] -> Logical Operator4/15
  [VDDM_ESC7RCErrCFS_flg] -> Logical Operator4/13
  [VDDM_ESC5RCErrCFS_flg] -> Logical Operator4/19
  [VDDM_ESC7CSErrCFS_flg] -> Logical Operator4/14
  [VDDM_BMSSigErrCFS_flg] -> Logical Operator4/1
  [VDDM_FrMCUSigErrCFS_flg] -> Logical Operator4/2
  [VDDM_RrMCUSigErrCFS_flg] -> Logical Operator4/3
  [VDDM_ZoneSCPNoComCFS_flg] -> Logical Operator4/5
  [VDDM_ESC1RCErrCFS_flg] -> Logical Operator4/16
  [VDDM_ESC5CSErrCFS_flg] -> Logical Operator14/20
  [VDDM_ESC5RCErrCFS_flg] -> Logical Operator14/19
  [VDDM_ESC5NoComCFS_flg] -> Logical Operator14/18
  [VDDM_ESC1CSErrCFS_flg] -> Logical Operator14/17
  [VDDM_ESC1RCErrCFS_flg] -> Logical Operator14/16
  [VDDM_ESC1NoComCFS_flg] -> Logical Operator14/15
  [VDDM_ESC7CSErrCFS_flg] -> Logical Operator14/14
  [VDDM_ESC7RCErrCFS_flg] -> Logical Operator14/13
  [VDDM_ESC7NoComCFS_flg] -> Logical Operator14/12
  [VDDM_MCUF1CSErrCFS_flg] -> Logical Operator14/11
  [VDDM_MCUF1RCErrCFS_flg] -> Logical Operator14/10
  [VDDM_MCUF1NoComCFS_flg] -> Logical Operator14/9
  [VDDM_MCUR1CSErrCFS_flg] -> Logical Operator14/8
  [VDDM_MCUR1RCErrCFS_flg] -> Logical Operator14/7
  [VDDM_MCUR1NoComCFS_flg] -> Logical Operator14/6
  [VDDM_ZoneSCPNoComCFS_flg] -> Logical Operator14/5
  [VDDM_CCUSigErrCFS_flg] -> Logical Operator14/4
  [VDDM_RrMCUSigErrCFS_flg] -> Logical Operator14/3
  [VDDM_FrMCUSigErrCFS_flg] -> Logical Operator14/2
  [VDDM_BMSSigErrCFS_flg] -> Logical Operator14/1
  Logical Operator1/1 -> Switch3/2
  [No_CAN1_BUS_OFF] -> Logical Operator1/1
  [No_CAN3_BUS_OFF] -> Logical Operator1/2
  Equal4/1 -> Logical Operator1/5
  Equal5/1 -> Logical Operator1/4
  Constant8/1 -> Equal5/2
  Constant10/1 -> Equal4/2
  [VPMM_PowerSta_enum] -> Equal5/1
  [No_CAN4_BUS_OFF] -> Logical Operator1/3
  [VINP_ZoneSpdCtrlMode_enum] -> Equal4/1
  Equal1/1 -> Logical Operator2/5
  Constant3/1 -> Equal1/2
  [VINP_ZoneSpdCtrlMode_enum] -> Equal1/1
  [VPMM_PowerSta_enum] -> Equal2/1
  Constant1/1 -> Equal2/2
  Equal2/1 -> Logical Operator2/4
  [No_CAN4_BUS_OFF] -> Logical Operator2/3
  [No_CAN3_BUS_OFF] -> Logical Operator2/2
  Logical Operator14/1 -> Switch2/1
  VDDM_ESC5RCErrCFS_flg/1 -> [VDDM_ESC5RCErrCFS_flg]
  VDDM_ESC5CSErrCFS_flg/1 -> [VDDM_ESC5CSErrCFS_flg]
  VDDM_ESC5NoComCFS_flg/1 -> [VDDM_ESC5NoComCFS_flg]
  VDDM_ZoneSCPNoComCFS_flg/1 -> [VDDM_ZoneSCPNoComCFS_flg]
  task_time_s/1 -> [task_time_s]  "task_time_s"
  VINP_ZoneSpdCtrlMode_enum/1 -> [VINP_ZoneSpdCtrlMode_enum]
  No_CAN3_BUS_OFF/1 -> [No_CAN3_BUS_OFF]
  No_CAN1_BUS_OFF/1 -> [No_CAN1_BUS_OFF]
  VDDM_BMSSigErrCFS_flg/1 -> [VDDM_BMSSigErrCFS_flg]
  VDDM_ESC7NoComCFS_flg/1 -> [VDDM_ESC7NoComCFS_flg]
  VDDM_ESC7CSErrCFS_flg/1 -> [VDDM_ESC7CSErrCFS_flg]
  VPMM_PowerSta_enum/1 -> [VPMM_PowerSta_enum]
  No_CAN4_BUS_OFF/1 -> [No_CAN4_BUS_OFF]
  VDDM_ESC7RCErrCFS_flg/1 -> [VDDM_ESC7RCErrCFS_flg]
  VDDM_RrMCUSigErrCFS_flg/1 -> [VDDM_RrMCUSigErrCFS_flg]
  VDDM_CCUSigErrCFS_flg/1 -> [VDDM_CCUSigErrCFS_flg]
  VDDM_FrMCUSigErrCFS_flg/1 -> [VDDM_FrMCUSigErrCFS_flg]
  VDDM_MCUF1RCErrCFS_flg/1 -> [VDDM_MCUF1RCErrCFS_flg]
  VDDM_ESC1NoComCFS_flg/1 -> [VDDM_ESC1NoComCFS_flg]
  DTC_clear_request/1 -> [DTC_clear_request]
  VDDM_MCUR1RCErrCFS_flg/1 -> [VDDM_MCUR1RCErrCFS_flg]
  VDDM_MCUR1CSErrCFS_flg/1 -> [VDDM_MCUR1CSErrCFS_flg]
  VDDM_ESC1RCErrCFS_flg/1 -> [VDDM_ESC1RCErrCFS_flg]
  VDDM_ESC1CSErrCFS_flg/1 -> [VDDM_ESC1CSErrCFS_flg]
  VDDM_MCUF1CSErrCFS_flg/1 -> [VDDM_MCUF1CSErrCFS_flg]
  VDDM_MCUF1NoComCFS_flg/1 -> [VDDM_MCUF1NoComCFS_flg]
  VDDM_MCUR1NoComCFS_flg/1 -> [VDDM_MCUR1NoComCFS_flg]
  [VDDM_CCMalfuncPass_flg] -> Logical Operator12/1
  Constant12/1 -> Equal6/2
  Constant13/1 -> Equal7/2
  Equal6/1 -> Logical Operator13/1
  Logical Operator13/1 -> Logical Operator12/2
  Equal7/1 -> Logical Operator13/2
  Unit Delay2/1 -> Equal6/1
  [VPMM_PowerSta_enum] -> Equal7/1
  [VPMM_PowerSta_enum] -> Unit Delay2/1
  Constant9/1 -> Timer1/4
  Gain1/1 -> Timer1/3
  Test Detection Criteria/1 -> [VDDM_CCMalfuncDet_flg]  "VDDM_CCMalfuncDet_flg"
  Constant7/1 -> Test Detection Criteria/3
  Gain/1 -> Test Detection Criteria/4
  Constant4/1 -> Gain/1
  [task_time_s] -> Test Detection Criteria/2
  Switch3/1 -> Logical Operator6/1, Timer1/2
  Constant5/1 -> Switch3/3
  Timer1/1 -> Equal3/1
  Logical Operator12/1 -> Switch4/2
  Constant14/1 -> Switch4/1
  Constant2/1 -> Switch2/3
  Logical Operator6/1 -> Timer1/1
  Logical Operator2/1 -> Switch2/2
  [DTC_clear_request] -> Logical Operator12/3
  [VDDM_xxx_flg] -> SR_Latch1/2
  [No_CAN1_BUS_OFF] -> Logical Operator2/1
  Switch4/1 -> [VDDM_CCMalfuncCFSRls_flg]  "VDDM_CCMalfuncCFSRls_flg"
  Constant6/1 -> Equal3/2
  [task_time_s] -> Gain1/1
  Equal3/1 -> SR_Latch1/1
  Constant15/1 -> Switch4/3
  [VDDM_CCMalfuncCFS_flg] -> VDDM_CCMalfuncCFS_flg/1
  From1/1 -> Terminator1/1
  SR_Latch1/1 -> [VDDM_CCMalfuncPass_flg]  "VDDM_CCMalfuncPass_flg"
  [VDDM_CCMalfuncPass_flg] -> Switch1/2
  [VDDM_CCMalfuncCFS_flg] -> Switch/2
  Constant18/1 -> Switch/1
  Switch/1 -> Goto7/1
  Constant21/1 -> Switch/3
  Switch1/1 -> [VDDM_CCMalfuncDFSRls_flg]
  Constant22/1 -> Switch1/1
  Constant23/1 -> Switch1/3
